simulink model "ASM_Traffic_V2X_Complete_Model_2"  (R2019a)
settings: Solver=ode1  StartTime=SIM.tstart.v  StopTime=Inf  FixedStep=SIM.StepSize.v  RelTol=1e-3
PostLoadFcn:
  | if any(exist('dsrtsu_mdlpostloadfcn', 'file') ~= 0), dsrtsu_mdlpostloadfcn('Execute', bdroot); end
  | try, asm_mdl_postloadfcn(bdroot, 'UpdateModel', 2200); catch, disp(lasterr); end,
undefined symbols (not defined in the file): _SensorPnts_1, _SensorPnts_13, _SensorPnts_17, _SensorPnts_21, _SensorPnts_25, _SensorPnts_29, _SensorPnts_33, _SensorPnts_37, _SensorPnts_41, _SensorPnts_45, _SensorPnts_49, _SensorPnts_5, _SensorPnts_53, _SensorPnts_57, _SensorPnts_9, _to_, CPT, G5A, ITS, MDL, rad, s_to_rpm, SIM
libraries: simulink x169, ASM_VehicleDynamics_lib x126, ASM_Traffic_lib x83, ASM_Utils_lib x49, mdbs x45, ASM_Environment_lib x17, dspindex x12, dsaV2xLibraryAux x10, dsmpblib x6, dsaV2xAsn1Library x4, dsaV2xLibrary x4, ASM_BrakeHydraulics_lib x4
(part 17 of 36)

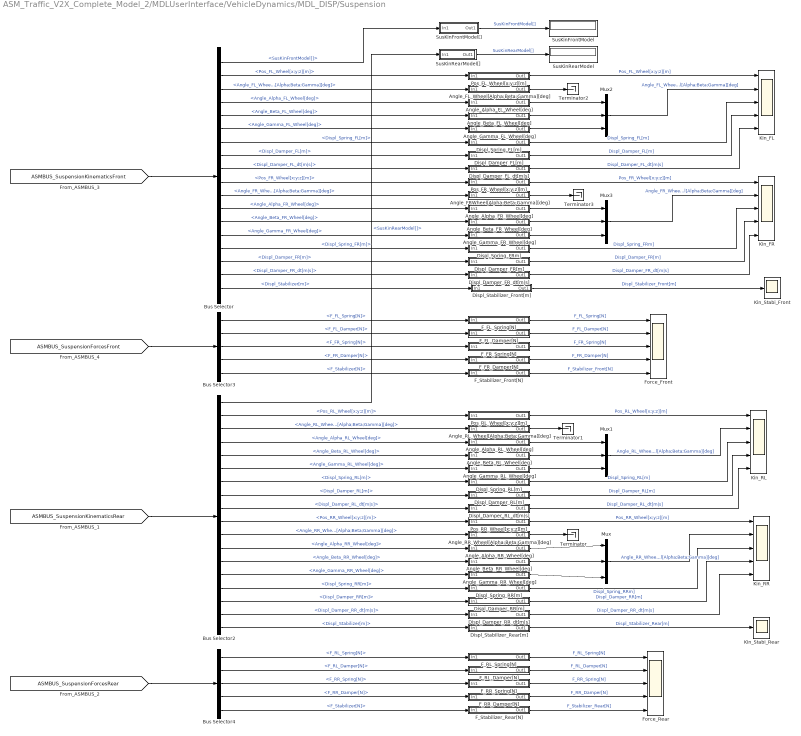
== system ASM_Traffic_V2X_Complete_Model_2/MDLUserInterface/VehicleDynamics/MDL_DISP/Suspension ==
  Angle_Alpha_FL_Wheel[deg] : Subsystem
      mask Display: disp('')
  Angle_Alpha_FR_Wheel[deg] : Subsystem
      mask Display: disp('')
  Angle_Alpha_RL_Wheel[deg] : Subsystem
      mask Display: disp('')
  Angle_Alpha_RR_Wheel[deg] : Subsystem
      mask Display: disp('')
  Angle_Beta_FL_Wheel[deg] : Subsystem
      mask Display: disp('')
  Angle_Beta_FR_Wheel[deg] : Subsystem
      mask Display: disp('')
  Angle_Beta_RL_Wheel[deg] : Subsystem
      mask Display: disp('')
  Angle_Beta_RR_Wheel[deg] : Subsystem
      mask Display: disp('')
  Angle_FL_Wheel[Alpha;Beta;Gamma][deg] : Subsystem
      mask Display: disp('')
  Angle_FRWheel[Alpha;Beta;Gamma][deg] : Subsystem
      mask Display: disp('')
  Angle_Gamma_FL_Wheel[deg] : Subsystem
      mask Display: disp('')
  Angle_Gamma_FR_Wheel[deg] : Subsystem
      mask Display: disp('')
  Angle_Gamma_RL_Wheel[deg] : Subsystem
      mask Display: disp('')
  Angle_Gamma_RR_Wheel[deg] : Subsystem
      mask Display: disp('')
  Angle_RL_Wheel[Alpha;Beta;Gamma][deg] : Subsystem
      mask Display: disp('')
  Angle_RR_Wheel[Alpha;Beta;Gamma][deg] : Subsystem
      mask Display: disp('')
  Bus Selector : BusSelector  OutputSignals=SusKinFrontModel[],Kinematics_Left.Position_Left.Pos_FL_Wheel[x;y;z][m],Kinematics_Left.Orientation_Left.Angle_FL_Wheel[Alpha;Beta;Gamma][deg],Kinematics_Left.Orientation_Left.Angle_FL_Wheel[Alpha;Beta;Gamma][deg].Angle_Alpha_FL_Wheel[deg],Kinematics_Left.Orientation_Left.Angle_FL_Wheel[Alpha;Beta;Gamma][deg].Angle_Beta_FL_Wheel[deg],Kinematics_Left.Orientation_Left.Angle_FL_Wheel[Alpha;Beta;Gamma][deg].Angle_Gamma_FL_Wheel[deg],Kinematics_Left.Spring_Left.Displ_Spring_FL[m],Kinematics_Left.Damper_Left.Displ_Damper_FL[m],Kinematics_Left.Damper_Left.Displ_Damper_FL_dt[m|s],Kinematics_Right.Position_Right.Pos_FR_Wheel[x;y;z][m],Kinematics_Right.Orientation_Right.Angle_FR_Wheel[Alpha;Beta;Gamma][deg],Kinematics_Right.Orientation_Right.Angle_FR_Wheel[Alpha;Beta;Gamma][deg].Angle_Alpha_FR_Wheel[deg],Kinematics_Right.Orientation_Right.Angle_FR_Wheel[Alpha;Beta;Gamma][deg].Angle_Beta_FR_Wheel[deg],Kinematics_Right.Orientation_Right.Angle_FR_Wheel[Alpha;Beta;Gamma][deg].Angle_Gamma_FR_Wheel[deg],Kinematics_Right.Spring_Right.Displ_Spring_FR[m],Kinematics_Right.Damper_Right.Displ_Damper_FR[m],Kinematics_Right.Damper_Right.Displ_Damper_FR_dt[m|s],Stabilizer.Displ_Stabilizer[m]
  Bus Selector2 : BusSelector  OutputSignals=SusKinRearModel[],Kinematics_Left.Position_Left.Pos_RL_Wheel[x;y;z][m],Kinematics_Left.Orientation_Left.Angle_RL_Wheel[Alpha;Beta;Gamma][deg],Kinematics_Left.Orientation_Left.Angle_RL_Wheel[Alpha;Beta;Gamma][deg].Angle_Alpha_RL_Wheel[deg],Kinematics_Left.Orientation_Left.Angle_RL_Wheel[Alpha;Beta;Gamma][deg].Angle_Beta_RL_Wheel[deg],Kinematics_Left.Orientation_Left.Angle_RL_Wheel[Alpha;Beta;Gamma][deg].Angle_Gamma_RL_Wheel[deg],Kinematics_Left.Spring_Left.Displ_Spring_RL[m],Kinematics_Left.Damper_Left.Displ_Damper_RL[m],Kinematics_Left.Damper_Left.Displ_Damper_RL_dt[m|s],Kinematics_Right.Position_Right.Pos_RR_Wheel[x;y;z][m],Kinematics_Right.Orientation_Right.Angle_RR_Wheel[Alpha;Beta;Gamma][deg],Kinematics_Right.Orientation_Right.Angle_RR_Wheel[Alpha;Beta;Gamma][deg].Angle_Alpha_RR_Wheel[deg],Kinematics_Right.Orientation_Right.Angle_RR_Wheel[Alpha;Beta;Gamma][deg].Angle_Beta_RR_Wheel[deg],Kinematics_Right.Orientation_Right.Angle_RR_Wheel[Alpha;Beta;Gamma][deg].Angle_Gamma_RR_Wheel[deg],Kinematics_Right.Spring_Right.Displ_Spring_RR[m],Kinematics_Right.Damper_Right.Displ_Damper_RR[m],Kinematics_Right.Damper_Right.Displ_Damper_RR_dt[m|s],Stabilizer.Displ_Stabilizer[m]
  Bus Selector3 : BusSelector  OutputSignals=F_FL_Spring[N],F_FL_Damper[N],F_FR_Spring[N],F_FR_Damper[N],F_Stabilizer[N]
  Bus Selector4 : BusSelector  OutputSignals=F_RL_Spring[N],F_RL_Damper[N],F_RR_Spring[N],F_RR_Damper[N],F_Stabilizer[N]
  Displ_Damper_FL[m] : Subsystem
      mask Display: disp('')
  Displ_Damper_FL_dt[m|s] : Subsystem
      mask Display: disp('')
  Displ_Damper_FR[m] : Subsystem
      mask Display: disp('')
  Displ_Damper_FR_dt[m|s] : Subsystem
      mask Display: disp('')
  Displ_Damper_RL[m] : Subsystem
      mask Display: disp('')
  Displ_Damper_RL_dt[m|s] : Subsystem
      mask Display: disp('')
  Displ_Damper_RR[m] : Subsystem
      mask Display: disp('')
  Displ_Damper_RR_dt[m|s] : Subsystem
      mask Display: disp('')
  Displ_Spring_FL[m] : Subsystem
      mask Display: disp('')
  Displ_Spring_FRm] : Subsystem
      mask Display: disp('')
  Displ_Spring_RL[m] : Subsystem
      mask Display: disp('')
  Displ_Spring_RR[m] : Subsystem
      mask Display: disp('')
  Displ_Stabilizer_Front[m] : Subsystem
      mask Display: disp('')
  Displ_Stabilizer_Rear[m] : Subsystem
      mask Display: disp('')
  F_FL_Damper[N] : Subsystem
      mask Display: disp('')
  F_FL_Spring[N] : Subsystem
      mask Display: disp('')
  F_FR_Damper[N] : Subsystem
      mask Display: disp('')
  F_FR_Spring[N] : Subsystem
      mask Display: disp('')
  F_RL_Damper[N] : Subsystem
      mask Display: disp('')
  F_RL_Spring[N] : Subsystem
      mask Display: disp('')
  F_RR_Damper[N] : Subsystem
      mask Display: disp('')
  F_RR_Spring[N] : Subsystem
      mask Display: disp('')
  F_Stabilizer_Front[N] : Subsystem
      mask Display: disp('')
  F_Stabilizer_Rear[N] : Subsystem
      mask Display: disp('')
  Force_Front : Scope  NumInputPorts=5
  Force_Rear : Scope  NumInputPorts=5
  Kin_FL : Scope  NumInputPorts=5
  Kin_FR : Scope  NumInputPorts=5
  Kin_RL : Scope  NumInputPorts=5
  Kin_RR : Scope  NumInputPorts=5
  Kin_Stabi_Front : Scope
  Kin_Stabi_Rear : Scope
  Mux{,1..3} (4 alike) : Mux  Inputs=3
  Pos_FL_Wheel[x;y;z][m] : Subsystem
      mask Display: disp('')
  Pos_FR_Wheel[x;y;z][m] : Subsystem
      mask Display: disp('')
  Pos_RL_Wheel[x;y;z][m] : Subsystem
      mask Display: disp('')
  Pos_RR_Wheel[x;y;z][m] : Subsystem
      mask Display: disp('')
  SusKinFrontModel : Display
  SusKinFrontModel[] : Subsystem
      mask Display: disp('')
  SusKinRearModel : Display
  SusKinRearModel[] : Subsystem
      mask Display: disp('')
  Terminator{,1..3} (4 alike) : Terminator
  wires:
  Bus Selector/14 -> Angle_Gamma_FR_Wheel[deg]/1(In1)  "<Angle_Gamma_FR_Wheel[deg]>"
  Bus Selector/13 -> Angle_Beta_FR_Wheel[deg]/1(In1)  "<Angle_Beta_FR_Wheel[deg]>"
  Bus Selector/12 -> Angle_Alpha_FR_Wheel[deg]/1(In1)  "<Angle_Alpha_FR_Wheel[deg]>"
  Angle_FRWheel[Alpha;Beta;Gamma][deg]/1(Out1) -> Terminator3/1
  Mux3/1 -> Kin_FR/2  "Angle_FR_Wheel[Alpha;Beta;Gamma][deg]"
  Angle_Gamma_FR_Wheel[deg]/1(Out1) -> Mux3/3
  Angle_Beta_FR_Wheel[deg]/1(Out1) -> Mux3/2
  Angle_Alpha_FR_Wheel[deg]/1(Out1) -> Mux3/1
  Bus Selector/15 -> Displ_Spring_FRm]/1(In1)  "<Displ_Spring_FR[m]>"
  Bus Selector/16 -> Displ_Damper_FR[m]/1(In1)  "<Displ_Damper_FR[m]>"
  Bus Selector/17 -> Displ_Damper_FR_dt[m|s]/1(In1)  "<Displ_Damper_FR_dt[m|s]>"
  Bus Selector/18 -> Displ_Stabilizer_Front[m]/1(In1)  "<Displ_Stabilizer[m]>"
  Bus Selector/11 -> Angle_FRWheel[Alpha;Beta;Gamma][deg]/1(In1)  "<Angle_FR_Wheel[Alpha;Beta;Gamma][deg]>"
  Bus Selector/10 -> Pos_FR_Wheel[x;y;z][m]/1(In1)  "<Pos_FR_Wheel[x;y;z][m]>"
  Bus Selector/9 -> Displ_Damper_FL_dt[m|s]/1(In1)  "<Displ_Damper_FL_dt[m|s]>"
  Bus Selector/8 -> Displ_Damper_FL[m]/1(In1)  "<Displ_Damper_FL[m]>"
  Bus Selector/7 -> Displ_Spring_FL[m]/1(In1)  "<Displ_Spring_FL[m]>"
  Bus Selector/6 -> Angle_Gamma_FL_Wheel[deg]/1(In1)  "<Angle_Gamma_FL_Wheel[deg]>"
  Bus Selector/5 -> Angle_Beta_FL_Wheel[deg]/1(In1)  "<Angle_Beta_FL_Wheel[deg]>"
  Bus Selector/4 -> Angle_Alpha_FL_Wheel[deg]/1(In1)  "<Angle_Alpha_FL_Wheel[deg]>"
  Mux2/1 -> Kin_FL/2  "Angle_FL_Wheel[Alpha;Beta;Gamma][deg]"
  Angle_FL_Wheel[Alpha;Beta;Gamma][deg]/1(Out1) -> Terminator2/1
  Angle_Gamma_FL_Wheel[deg]/1(Out1) -> Mux2/3
  Angle_Beta_FL_Wheel[deg]/1(Out1) -> Mux2/2
  Angle_Alpha_FL_Wheel[deg]/1(Out1) -> Mux2/1
  Bus Selector/3 -> Angle_FL_Wheel[Alpha;Beta;Gamma][deg]/1(In1)  "<Angle_FL_Wheel[Alpha;Beta;Gamma][deg]>"
  Angle_RL_Wheel[Alpha;Beta;Gamma][deg]/1(Out1) -> Terminator1/1
  Bus Selector2/6 -> Angle_Gamma_RL_Wheel[deg]/1(In1)  "<Angle_Gamma_RL_Wheel[deg]>"
  Bus Selector2/5 -> Angle_Beta_RL_Wheel[deg]/1(In1)  "<Angle_Beta_RL_Wheel[deg]>"
  Bus Selector2/4 -> Angle_Alpha_RL_Wheel[deg]/1(In1)  "<Angle_Alpha_RL_Wheel[deg]>"
  Mux1/1 -> Kin_RL/2  "Angle_RL_Wheel[Alpha;Beta;Gamma][deg]"
  Angle_Gamma_RL_Wheel[deg]/1(Out1) -> Mux1/3
  Angle_Beta_RL_Wheel[deg]/1(Out1) -> Mux1/2
  Angle_Alpha_RL_Wheel[deg]/1(Out1) -> Mux1/1
  Angle_RR_Wheel[Alpha;Beta;Gamma][deg]/1(Out1) -> Terminator/1
  Mux/1 -> Kin_RR/2  "Angle_RR_Wheel[Alpha;Beta;Gamma][deg]"
  Angle_Gamma_RR_Wheel[deg]/1(Out1) -> Mux/3
  Angle_Beta_RR_Wheel[deg]/1(Out1) -> Mux/2
  Angle_Alpha_RR_Wheel[deg]/1(Out1) -> Mux/1
  Bus Selector2/14 -> Angle_Gamma_RR_Wheel[deg]/1(In1)  "<Angle_Gamma_RR_Wheel[deg]>"
  Bus Selector2/13 -> Angle_Beta_RR_Wheel[deg]/1(In1)  "<Angle_Beta_RR_Wheel[deg]>"
  Bus Selector2/12 -> Angle_Alpha_RR_Wheel[deg]/1(In1)  "<Angle_Alpha_RR_Wheel[deg]>"
  Bus Selector2/1 -> SusKinRearModel[]/1(In1)  "<SusKinRearModel[]>"
  Bus Selector/1 -> SusKinFrontModel[]/1(In1)  "<SusKinFrontModel[]>"
  Bus Selector2/2 -> Pos_RL_Wheel[x;y;z][m]/1(In1)  "<Pos_RL_Wheel[x;y;z][m]>"
  Bus Selector/2 -> Pos_FL_Wheel[x;y;z][m]/1(In1)  "<Pos_FL_Wheel[x;y;z][m]>"
  [ASMBUS_SuspensionForcesRear] -> Bus Selector4/1
  [ASMBUS_SuspensionKinematicsRear] -> Bus Selector2/1
  [ASMBUS_SuspensionForcesFront] -> Bus Selector3/1
  [ASMBUS_SuspensionKinematicsFront] -> Bus Selector/1
  Bus Selector4/5 -> F_Stabilizer_Rear[N]/1(In1)  "<F_Stabilizer[N]>"
  Bus Selector4/4 -> F_RR_Damper[N]/1(In1)  "<F_RR_Damper[N]>"
  Bus Selector4/3 -> F_RR_Spring[N]/1(In1)  "<F_RR_Spring[N]>"
  Bus Selector4/2 -> F_RL_Damper[N]/1(In1)  "<F_RL_Damper[N]>"
  Bus Selector4/1 -> F_RL_Spring[N]/1(In1)  "<F_RL_Spring[N]>"
  Bus Selector2/18 -> Displ_Stabilizer_Rear[m]/1(In1)  "<Displ_Stabilizer[m]>"
  Bus Selector2/17 -> Displ_Damper_RR_dt[m|s]/1(In1)  "<Displ_Damper_RR_dt[m|s]>"
  Bus Selector2/16 -> Displ_Damper_RR[m]/1(In1)  "<Displ_Damper_RR[m]>"
  Bus Selector2/15 -> Displ_Spring_RR[m]/1(In1)  "<Displ_Spring_RR[m]>"
  Bus Selector2/11 -> Angle_RR_Wheel[Alpha;Beta;Gamma][deg]/1(In1)  "<Angle_RR_Wheel[Alpha;Beta;Gamma][deg]>"
  Bus Selector2/10 -> Pos_RR_Wheel[x;y;z][m]/1(In1)  "<Pos_RR_Wheel[x;y;z][m]>"
  Bus Selector2/9 -> Displ_Damper_RL_dt[m|s]/1(In1)  "<Displ_Damper_RL_dt[m|s]>"
  Bus Selector2/8 -> Displ_Damper_RL[m]/1(In1)  "<Displ_Damper_RL[m]>"
  Bus Selector2/7 -> Displ_Spring_RL[m]/1(In1)  "<Displ_Spring_RL[m]>"
  Bus Selector2/3 -> Angle_RL_Wheel[Alpha;Beta;Gamma][deg]/1(In1)  "<Angle_RL_Wheel[Alpha;Beta;Gamma][deg]>"
  Displ_Damper_RR_dt[m|s]/1(Out1) -> Kin_RR/5  "Displ_Damper_RR_dt[m|s]"
  Displ_Damper_RR[m]/1(Out1) -> Kin_RR/4  "Displ_Damper_RR[m]"
  Displ_Spring_RR[m]/1(Out1) -> Kin_RR/3  "Displ_Spring_RRm]"
  Pos_RR_Wheel[x;y;z][m]/1(Out1) -> Kin_RR/1  "Pos_RR_Wheel[x;y;z][m]"
  Displ_Stabilizer_Rear[m]/1(Out1) -> Kin_Stabi_Rear/1  "Displ_Stabilizer_Rear[m]"
  F_RL_Spring[N]/1(Out1) -> Force_Rear/1  "F_RL_Spring[N]"
  F_RL_Damper[N]/1(Out1) -> Force_Rear/2  "F_RL_Damper[N]"
  F_Stabilizer_Rear[N]/1(Out1) -> Force_Rear/5  "F_Stabilizer_Rear[N]"
  F_RR_Damper[N]/1(Out1) -> Force_Rear/4  "F_RR_Damper[N]"
  F_RR_Spring[N]/1(Out1) -> Force_Rear/3  "F_RR_Spring[N]"
  Displ_Damper_RL_dt[m|s]/1(Out1) -> Kin_RL/5  "Displ_Damper_RL_dt[m|s]"
  Displ_Damper_RL[m]/1(Out1) -> Kin_RL/4  "Displ_Damper_RL[m]"
  Displ_Spring_RL[m]/1(Out1) -> Kin_RL/3  "Displ_Spring_RL[m]"
  Pos_RL_Wheel[x;y;z][m]/1(Out1) -> Kin_RL/1  "Pos_RL_Wheel[x;y;z][m]"
  Displ_Damper_FR_dt[m|s]/1(Out1) -> Kin_FR/5  "Displ_Damper_FR_dt[m|s]"
  Displ_Damper_FR[m]/1(Out1) -> Kin_FR/4  "Displ_Damper_FR[m]"
  Displ_Spring_FRm]/1(Out1) -> Kin_FR/3  "Displ_Spring_FRm]"
  Pos_FR_Wheel[x;y;z][m]/1(Out1) -> Kin_FR/1  "Pos_FR_Wheel[x;y;z][m]"
  Displ_Stabilizer_Front[m]/1(Out1) -> Kin_Stabi_Front/1  "Displ_Stabilizer_Front[m]"
  F_FL_Spring[N]/1(Out1) -> Force_Front/1  "F_FL_Spring[N]"
  F_FL_Damper[N]/1(Out1) -> Force_Front/2  "F_FL_Damper[N]"
  F_Stabilizer_Front[N]/1(Out1) -> Force_Front/5  "F_Stabilizer_Front[N]"
  F_FR_Damper[N]/1(Out1) -> Force_Front/4  "F_FR_Damper[N]"
  F_FR_Spring[N]/1(Out1) -> Force_Front/3  "F_FR_Spring[N]"
  Bus Selector3/5 -> F_Stabilizer_Front[N]/1(In1)  "<F_Stabilizer[N]>"
  Bus Selector3/4 -> F_FR_Damper[N]/1(In1)  "<F_FR_Damper[N]>"
  Bus Selector3/3 -> F_FR_Spring[N]/1(In1)  "<F_FR_Spring[N]>"
  Bus Selector3/2 -> F_FL_Damper[N]/1(In1)  "<F_FL_Damper[N]>"
  Bus Selector3/1 -> F_FL_Spring[N]/1(In1)  "<F_FL_Spring[N]>"
  SusKinRearModel[]/1(Out1) -> SusKinRearModel/1  "SusKinRearModel[]"
  SusKinFrontModel[]/1(Out1) -> SusKinFrontModel/1  "SusKinFrontModel[]"
  Displ_Damper_FL_dt[m|s]/1(Out1) -> Kin_FL/5  "Displ_Damper_FL_dt[m|s]"
  Displ_Damper_FL[m]/1(Out1) -> Kin_FL/4  "Displ_Damper_FL[m]"
  Displ_Spring_FL[m]/1(Out1) -> Kin_FL/3  "Displ_Spring_FL[m]"
  Pos_FL_Wheel[x;y;z][m]/1(Out1) -> Kin_FL/1  "Pos_FL_Wheel[x;y;z][m]"

== system ASM_Traffic_V2X_Complete_Model_2/MDLUserInterface/VehicleDynamics/MDL_DISP/Tire ==
  Tire : Inport
  Bus Selector2 : BusSelector  OutputSignals=Tire_FL.ActiveTire.Slip_x_FL[],Tire_FR.ActiveTire.Slip_x_FR[],Tire_RL.ActiveTire.Slip_x_RL[],Tire_RR.ActiveTire.Slip_x_RR[],Tire_FL.ActiveTire.Slip_y_FL[],Tire_FR.ActiveTire.Slip_y_FR[],Tire_RL.ActiveTire.Slip_y_RL[],Tire_RR.ActiveTire.Slip_y_RR[],Tire_FL.ActiveTire.r_Dyn_FL_Tire[m],Tire_FR.ActiveTire.r_Dyn_FR_Tire[m],Tire_RL.ActiveTire.r_Dyn_RL_Tire[m],Tire_RR.ActiveTire.r_Dyn_RR_Tire[m],Tire_FL.ActiveTire.F_x_Dyn_FL_Tire_CoorSys_CP[N],Tire_FR.ActiveTire.F_x_Dyn_FR_Tire_CoorSys_CP[N],Tire_RL.ActiveTire.F_x_Dyn_RL_Tire_CoorSys_CP[N],Tire_RR.ActiveTire.F_x_Dyn_RR_Tire_CoorSys_CP[N],Tire_FL.ActiveTire.F_y_Dyn_FL_Tire_CoorSys_CP[N],Tire_FR.ActiveTire.F_y_Dyn_FR_Tire_CoorSys_CP[N],Tire_RL.ActiveTire.F_y_Dyn_RL_Tire_CoorSys_CP[N],Tire_RR.ActiveTire.F_y_Dyn_RR_Tire_CoorSys_CP[N],Tire_FL.ActiveTire.F_z_Dyn_FL_Tire_CoorSys_CP[N],Tire_FR.ActiveTire.F_z_Dyn_FR_Tire_CoorSys_CP[N],Tire_RL.ActiveTire.F_z_Dyn_RL_Tire_CoorSys_CP[N],Tire_RR.ActiveTire.F_z_Dyn_RR_Tire_CoorSys_CP[N],Tire_FL.ActiveTire.Trq_x_FL_CoorSys_CP[Nm],Tire_FR.ActiveTire.Trq_x_FR_CoorSys_CP[Nm],Tire_RL.ActiveTire.Trq_x_RL_CoorSys_CP[Nm],Tire_RR.ActiveTire.Trq_x_RR_CoorSys_CP[Nm],Tire_FL.ActiveTire.Trq_y_FL_CoorSys_W[Nm],Tire_FR.ActiveTire.Trq_y_FR_CoorSys_W[Nm],Tire_RL.ActiveTire.Trq_y_RL_CoorSys_W[Nm],Tire_RR.ActiveTire.Trq_y_RR_CoorSys_W[Nm],Tire_FL.ActiveTire.Trq_z_FL_CoorSys_CP[Nm],Tire_FR.ActiveTire.Trq_z_FR_CoorSys_CP[Nm],Tire_RL.ActiveTire.Trq_z_RL_CoorSys_CP[Nm],Tire_RR.ActiveTire.Trq_z_RR_CoorSys_CP[Nm],Tire_FL.ActiveTire.v_Circumf_Dyn_FL_Wheel[km|h],Tire_FR.ActiveTire.v_Circumf_Dyn_FR_Wheel[km|h],Tire_RL.ActiveTire.v_Circumf_Dyn_RL_Wheel[km|h],Tire_RR.ActiveTire.v_Circumf_Dyn_RR_Wheel[km|h]
  DynamicRadius : Scope  NumInputPorts=4
  F_x_Dyn_FL_Tire_CoorSys_CP[N] : Subsystem
      mask Display: disp('')
  F_x_Dyn_FR_Tire_CoorSys_CP[N] : Subsystem
      mask Display: disp('')
  F_x_Dyn_RL_Tire_CoorSys_CP[N] : Subsystem
      mask Display: disp('')
  F_x_Dyn_RR_Tire_CoorSys_CP[N] : Subsystem
      mask Display: disp('')
  F_y_Dyn_FL_Tire_CoorSys_CP[N] : Subsystem
      mask Display: disp('')
  F_y_Dyn_FR_Tire_CoorSys_CP[N] : Subsystem
      mask Display: disp('')
  F_y_Dyn_RL_Tire_CoorSys_CP[N] : Subsystem
      mask Display: disp('')
  F_y_Dyn_RR_Tire_CoorSys_CP[N] : Subsystem
      mask Display: disp('')
  F_z_Dyn_FL_Tire_CoorSys_CP[N] : Subsystem
      mask Display: disp('')
  F_z_Dyn_FR_Tire_CoorSys_CP[N] : Subsystem
      mask Display: disp('')
  F_z_Dyn_RL_Tire_CoorSys_CP[N] : Subsystem
      mask Display: disp('')
  F_z_Dyn_RR_Tire_CoorSys_CP[N] : Subsystem
      mask Display: disp('')
  Mux{,1..7} (8 alike) : Mux
  Slip : Scope  NumInputPorts=2
  Slip_x_FL[] : Subsystem
      mask Display: disp('')
  Slip_x_FR[] : Subsystem
      mask Display: disp('')
  Slip_x_RL[] : Subsystem
      mask Display: disp('')
  Slip_x_RR[] : Subsystem
      mask Display: disp('')
  Slip_y_FL[] : Subsystem
      mask Display: disp('')
  Slip_y_FR[] : Subsystem
      mask Display: disp('')
  Slip_y_RL[] : Subsystem
      mask Display: disp('')
  Slip_y_RR[] : Subsystem
      mask Display: disp('')
  TireCircumfSpeed : Scope  NumInputPorts=4
  TireForce : Scope  NumInputPorts=3
  TireTorque : Scope  NumInputPorts=3
  Trq_x_FL_CoorSys_CP[Nm] : Subsystem
      mask Display: disp('')
  Trq_x_FR_CoorSys_CP[Nm] : Subsystem
      mask Display: disp('')
  Trq_x_RL_CoorSys_CP[Nm] : Subsystem
      mask Display: disp('')
  Trq_x_RR_CoorSys_CP[Nm] : Subsystem
      mask Display: disp('')
  Trq_y_FL_CoorSys_W[Nm] : Subsystem
      mask Display: disp('')
  Trq_y_FR_CoorSys_W[Nm] : Subsystem
      mask Display: disp('')
  Trq_y_RL_CoorSys_W[Nm] : Subsystem
      mask Display: disp('')
  Trq_y_RR_CoorSys_W[Nm] : Subsystem
      mask Display: disp('')
  Trq_z_FL_CoorSys_CP[Nm] : Subsystem
      mask Display: disp('')
  Trq_z_FR_CoorSys_CP[Nm] : Subsystem
      mask Display: disp('')
  Trq_z_RL_CoorSys_CP[Nm] : Subsystem
      mask Display: disp('')
  Trq_z_RR_CoorSys_CP[Nm] : Subsystem
      mask Display: disp('')
  r_Dyn_FL_Tire[m] : Subsystem
      mask Display: disp('')
  r_Dyn_FR_Tire[m] : Subsystem
      mask Display: disp('')
  r_Dyn_RL_Tire[m] : Subsystem
      mask Display: disp('')
  r_Dyn_RR_Tire[m] : Subsystem
      mask Display: disp('')
  v_Circumf_Dyn_FL_Wheel[km|h] : Subsystem
      mask Display: disp('')
  v_Circumf_Dyn_FR_Wheel[km|h] : Subsystem
      mask Display: disp('')
  v_Circumf_Dyn_RL_Wheel[km|h] : Subsystem
      mask Display: disp('')
  v_Circumf_Dyn_RR_Wheel[km|h] : Subsystem
      mask Display: disp('')
  wires:
  Mux7/1 -> Slip/2  "Slip_y[]"
  Mux6/1 -> Slip/1  "Slip_x[]"
  Mux5/1 -> TireTorque/3  "Trq_z[Nm]"
  Mux3/1 -> TireTorque/2  "Trq_y[Nm]"
  Mux4/1 -> TireTorque/1  "Trq_x[Nm]"
  Mux2/1 -> TireForce/3  "F_z[N]"
  Mux/1 -> TireForce/2  "F_y[N]"
  Mux1/1 -> TireForce/1  "F_x[N]"
  Tire/1 -> Bus Selector2/1
  Slip_x_FL[]/1(Out1) -> Mux6/1  "Slip_x_FL[]"
  Slip_x_FR[]/1(Out1) -> Mux6/2  "Slip_x_FR[]"
  Slip_x_RL[]/1(Out1) -> Mux6/3  "Slip_x_RL[]"
  Slip_x_RR[]/1(Out1) -> Mux6/4  "Slip_x_RR[]"
  Slip_y_FL[]/1(Out1) -> Mux7/1  "Slip_y_FL[]"
  Slip_y_FR[]/1(Out1) -> Mux7/2  "Slip_y_FR[]"
  Slip_y_RL[]/1(Out1) -> Mux7/3  "Slip_y_RL[]"
  Slip_y_RR[]/1(Out1) -> Mux7/4  "Slip_y_RR[]"
  Bus Selector2/1 -> Slip_x_FL[]/1(In1)  "<Slip_x_FL[]>"
  Bus Selector2/2 -> Slip_x_FR[]/1(In1)  "<Slip_x_FR[]>"
  Bus Selector2/3 -> Slip_x_RL[]/1(In1)  "<Slip_x_RL[]>"
  Bus Selector2/4 -> Slip_x_RR[]/1(In1)  "<Slip_x_RR[]>"
  Bus Selector2/5 -> Slip_y_FL[]/1(In1)  "<Slip_y_FL[]>"
  Bus Selector2/6 -> Slip_y_FR[]/1(In1)  "<Slip_y_FR[]>"
  Bus Selector2/7 -> Slip_y_RL[]/1(In1)  "<Slip_y_RL[]>"
  Bus Selector2/8 -> Slip_y_RR[]/1(In1)  "<Slip_y_RR[]>"
  Trq_x_FL_CoorSys_CP[Nm]/1(Out1) -> Mux4/1  "Trq_x_FL_CoorSys_CP[Nm]"
  Trq_x_FR_CoorSys_CP[Nm]/1(Out1) -> Mux4/2  "Trq_x_FR_CoorSys_CP[Nm]"
  Trq_x_RL_CoorSys_CP[Nm]/1(Out1) -> Mux4/3  "Trq_x_RL_CoorSys_CP[Nm]"
  Trq_x_RR_CoorSys_CP[Nm]/1(Out1) -> Mux4/4  "Trq_x_RR_CoorSys_CP[Nm]"
  Trq_y_FL_CoorSys_W[Nm]/1(Out1) -> Mux3/1  "Trq_y_FL_CoorSys_W[Nm]"
  Trq_y_FR_CoorSys_W[Nm]/1(Out1) -> Mux3/2  "Trq_y_FR_CoorSys_W[Nm]"
  Trq_y_RL_CoorSys_W[Nm]/1(Out1) -> Mux3/3  "Trq_y_RL_CoorSys_W[Nm]"
  Trq_y_RR_CoorSys_W[Nm]/1(Out1) -> Mux3/4  "Trq_y_RR_CoorSys_W[Nm]"
  Trq_z_FL_CoorSys_CP[Nm]/1(Out1) -> Mux5/1  "Trq_z_FL_CoorSys_CP[Nm]"
  Trq_z_FR_CoorSys_CP[Nm]/1(Out1) -> Mux5/2  "Trq_z_FR_CoorSys_CP[Nm]"
  Trq_z_RL_CoorSys_CP[Nm]/1(Out1) -> Mux5/3  "Trq_z_RL_CoorSys_CP[Nm]"
  Trq_z_RR_CoorSys_CP[Nm]/1(Out1) -> Mux5/4  "Trq_z_RR_CoorSys_CP[Nm]"
  F_x_Dyn_FL_Tire_CoorSys_CP[N]/1(Out1) -> Mux1/1  "F_x_Dyn_FL_Tire_CoorSys_CP[N]"
  F_x_Dyn_FR_Tire_CoorSys_CP[N]/1(Out1) -> Mux1/2  "F_x_Dyn_FR_Tire_CoorSys_CP[N]"
  F_x_Dyn_RL_Tire_CoorSys_CP[N]/1(Out1) -> Mux1/3  "F_x_Dyn_RL_Tire_CoorSys_CP[N]"
  F_x_Dyn_RR_Tire_CoorSys_CP[N]/1(Out1) -> Mux1/4  "F_x_Dyn_RR_Tire_CoorSys_CP[N]"
  F_y_Dyn_FL_Tire_CoorSys_CP[N]/1(Out1) -> Mux/1  "F_y_Dyn_FL_Tire_CoorSys_CP[N]"
  F_y_Dyn_FR_Tire_CoorSys_CP[N]/1(Out1) -> Mux/2  "F_y_Dyn_FR_Tire_CoorSys_CP[N]"
  F_y_Dyn_RL_Tire_CoorSys_CP[N]/1(Out1) -> Mux/3  "F_y_Dyn_RL_Tire_CoorSys_CP[N]"
  F_y_Dyn_RR_Tire_CoorSys_CP[N]/1(Out1) -> Mux/4  "F_y_Dyn_RR_Tire_CoorSys_CP[N]"
  F_z_Dyn_FL_Tire_CoorSys_CP[N]/1(Out1) -> Mux2/1  "F_z_Dyn_FL_Tire_CoorSys_CP[N]"
  F_z_Dyn_FR_Tire_CoorSys_CP[N]/1(Out1) -> Mux2/2  "F_z_Dyn_FR_Tire_CoorSys_CP[N]"
  F_z_Dyn_RL_Tire_CoorSys_CP[N]/1(Out1) -> Mux2/3  "F_z_Dyn_RL_Tire_CoorSys_CP[N]"
  F_z_Dyn_RR_Tire_CoorSys_CP[N]/1(Out1) -> Mux2/4  "F_z_Dyn_RR_Tire_CoorSys_CP[N]"
  v_Circumf_Dyn_FL_Wheel[km|h]/1(Out1) -> TireCircumfSpeed/1  "v_Circumf_Dyn_FL_Wheel[km|h]"
  v_Circumf_Dyn_FR_Wheel[km|h]/1(Out1) -> TireCircumfSpeed/2  "v_Circumf_Dyn_FR_Wheel[km|h]"
  v_Circumf_Dyn_RL_Wheel[km|h]/1(Out1) -> TireCircumfSpeed/3  "v_Circumf_Dyn_RL_Wheel[km|h]"
  v_Circumf_Dyn_RR_Wheel[km|h]/1(Out1) -> TireCircumfSpeed/4  "v_Circumf_Dyn_RR_Wheel[km|h]"
  r_Dyn_FL_Tire[m]/1(Out1) -> DynamicRadius/1  "r_Dyn_FL_Tire[m]"
  r_Dyn_FR_Tire[m]/1(Out1) -> DynamicRadius/2  "r_Dyn_FR_Tire[m]"
  r_Dyn_RL_Tire[m]/1(Out1) -> DynamicRadius/3  "r_Dyn_RL_Tire[m]"
  r_Dyn_RR_Tire[m]/1(Out1) -> DynamicRadius/4  "r_Dyn_RR_Tire[m]"
  Bus Selector2/9 -> r_Dyn_FL_Tire[m]/1(In1)  "<r_Dyn_FL_Tire[m]>"
  Bus Selector2/10 -> r_Dyn_FR_Tire[m]/1(In1)  "<r_Dyn_FR_Tire[m]>"
  Bus Selector2/11 -> r_Dyn_RL_Tire[m]/1(In1)  "<r_Dyn_RL_Tire[m]>"
  Bus Selector2/12 -> r_Dyn_RR_Tire[m]/1(In1)  "<r_Dyn_RR_Tire[m]>"
  Bus Selector2/13 -> F_x_Dyn_FL_Tire_CoorSys_CP[N]/1(In1)  "<F_x_Dyn_FL_Tire_CoorSys_CP[N]>"
  Bus Selector2/14 -> F_x_Dyn_FR_Tire_CoorSys_CP[N]/1(In1)  "<F_x_Dyn_FR_Tire_CoorSys_CP[N]>"
  Bus Selector2/15 -> F_x_Dyn_RL_Tire_CoorSys_CP[N]/1(In1)  "<F_x_Dyn_RL_Tire_CoorSys_CP[N]>"
  Bus Selector2/16 -> F_x_Dyn_RR_Tire_CoorSys_CP[N]/1(In1)  "<F_x_Dyn_RR_Tire_CoorSys_CP[N]>"
  Bus Selector2/17 -> F_y_Dyn_FL_Tire_CoorSys_CP[N]/1(In1)  "<F_y_Dyn_FL_Tire_CoorSys_CP[N]>"
  Bus Selector2/18 -> F_y_Dyn_FR_Tire_CoorSys_CP[N]/1(In1)  "<F_y_Dyn_FR_Tire_CoorSys_CP[N]>"
  Bus Selector2/19 -> F_y_Dyn_RL_Tire_CoorSys_CP[N]/1(In1)  "<F_y_Dyn_RL_Tire_CoorSys_CP[N]>"
  Bus Selector2/20 -> F_y_Dyn_RR_Tire_CoorSys_CP[N]/1(In1)  "<F_y_Dyn_RR_Tire_CoorSys_CP[N]>"
  Bus Selector2/21 -> F_z_Dyn_FL_Tire_CoorSys_CP[N]/1(In1)  "<F_z_Dyn_FL_Tire_CoorSys_CP[N]>"
  Bus Selector2/22 -> F_z_Dyn_FR_Tire_CoorSys_CP[N]/1(In1)  "<F_z_Dyn_FR_Tire_CoorSys_CP[N]>"
  Bus Selector2/23 -> F_z_Dyn_RL_Tire_CoorSys_CP[N]/1(In1)  "<F_z_Dyn_RL_Tire_CoorSys_CP[N]>"
  Bus Selector2/24 -> F_z_Dyn_RR_Tire_CoorSys_CP[N]/1(In1)  "<F_z_Dyn_RR_Tire_CoorSys_CP[N]>"
  Bus Selector2/25 -> Trq_x_FL_CoorSys_CP[Nm]/1(In1)  "<Trq_x_FL_CoorSys_CP[Nm]>"
  Bus Selector2/26 -> Trq_x_FR_CoorSys_CP[Nm]/1(In1)  "<Trq_x_FR_CoorSys_CP[Nm]>"
  Bus Selector2/27 -> Trq_x_RL_CoorSys_CP[Nm]/1(In1)  "<Trq_x_RL_CoorSys_CP[Nm]>"
  Bus Selector2/28 -> Trq_x_RR_CoorSys_CP[Nm]/1(In1)  "<Trq_x_RR_CoorSys_CP[Nm]>"
  Bus Selector2/29 -> Trq_y_FL_CoorSys_W[Nm]/1(In1)  "<Trq_y_FL_CoorSys_W[Nm]>"
  Bus Selector2/30 -> Trq_y_FR_CoorSys_W[Nm]/1(In1)  "<Trq_y_FR_CoorSys_W[Nm]>"
  Bus Selector2/31 -> Trq_y_RL_CoorSys_W[Nm]/1(In1)  "<Trq_y_RL_CoorSys_W[Nm]>"
  Bus Selector2/32 -> Trq_y_RR_CoorSys_W[Nm]/1(In1)  "<Trq_y_RR_CoorSys_W[Nm]>"
  Bus Selector2/33 -> Trq_z_FL_CoorSys_CP[Nm]/1(In1)  "<Trq_z_FL_CoorSys_CP[Nm]>"
  Bus Selector2/34 -> Trq_z_FR_CoorSys_CP[Nm]/1(In1)  "<Trq_z_FR_CoorSys_CP[Nm]>"
  Bus Selector2/35 -> Trq_z_RL_CoorSys_CP[Nm]/1(In1)  "<Trq_z_RL_CoorSys_CP[Nm]>"
  Bus Selector2/36 -> Trq_z_RR_CoorSys_CP[Nm]/1(In1)  "<Trq_z_RR_CoorSys_CP[Nm]>"
  Bus Selector2/37 -> v_Circumf_Dyn_FL_Wheel[km|h]/1(In1)  "<v_Circumf_Dyn_FL_Wheel[km|h]>"
  Bus Selector2/38 -> v_Circumf_Dyn_FR_Wheel[km|h]/1(In1)  "<v_Circumf_Dyn_FR_Wheel[km|h]>"
  Bus Selector2/39 -> v_Circumf_Dyn_RL_Wheel[km|h]/1(In1)  "<v_Circumf_Dyn_RL_Wheel[km|h]>"
  Bus Selector2/40 -> v_Circumf_Dyn_RR_Wheel[km|h]/1(In1)  "<v_Circumf_Dyn_RR_Wheel[km|h]>"

== system ASM_Traffic_V2X_Complete_Model_2/MDLUserInterface/VehicleDynamics/MDL_DISP/Velocities ==
  Velocities : Inport
  Angle_SideSlip_Vehicle[deg] : Subsystem
      mask Display: disp('')
  AngularVelocities : Scope  NumInputPorts=3
  Bus Selector2 : BusSelector  OutputSignals=Vehicle.Linear.v_Vehicle_CoG[x;y;z][km|h].v_x_Vehicle_CoG[km|h],Vehicle.Linear.v_Vehicle_CoG[x;y;z][km|h].v_y_Vehicle_CoG[km|h],Vehicle.Linear.v_Vehicle_CoG[x;y;z][km|h].v_z_Vehicle_CoG[km|h],Vehicle.Linear.Angle_SideSlip_Vehicle[deg],Vehicle.Angular.w_Vehicle_CoG[x;y;z][deg|s].RollRate_Vehicle_CoG[deg|s],Vehicle.Angular.w_Vehicle_CoG[x;y;z][deg|s].PitchRate_Vehicle_CoG[deg|s],Vehicle.Angular.w_Vehicle_CoG[x;y;z][deg|s].YawRate_Vehicle_CoG[deg|s]
  PitchRate_Vehicle_CoG[deg|s] : Subsystem
      mask Display: disp('')
  RollRate_Vehicle_CoG[deg|s] : Subsystem
      mask Display: disp('')
  TransVelocities : Scope  NumInputPorts=4
  YawRate_Vehicle_CoG[deg|s] : Subsystem
      mask Display: disp('')
  v_x_Vehicle_CoG[km|h] : Subsystem
      mask Display: disp('')
  v_y_Vehicle_CoG[km|h] : Subsystem
      mask Display: disp('')
  v_z_Vehicle_CoG[km|h] : Subsystem
      mask Display: disp('')
  wires:
  Velocities/1 -> Bus Selector2/1
  RollRate_Vehicle_CoG[deg|s]/1(Out1) -> AngularVelocities/1  "RollRate_Vehicle_CoG[deg|s]"
  PitchRate_Vehicle_CoG[deg|s]/1(Out1) -> AngularVelocities/2  "PitchRate_Vehicle_CoG[deg|s]"
  YawRate_Vehicle_CoG[deg|s]/1(Out1) -> AngularVelocities/3  "YawRate_Vehicle_CoG[deg|s]"
  v_x_Vehicle_CoG[km|h]/1(Out1) -> TransVelocities/1  "v_x_Vehicle_CoG[km|h]"
  v_y_Vehicle_CoG[km|h]/1(Out1) -> TransVelocities/2  "v_y_Vehicle_CoG[km|h]"
  v_z_Vehicle_CoG[km|h]/1(Out1) -> TransVelocities/3  "v_z_Vehicle_CoG[km|h]"
  Angle_SideSlip_Vehicle[deg]/1(Out1) -> TransVelocities/4  "Angle_SideSlip_Vehicle[deg]"
  Bus Selector2/1 -> v_x_Vehicle_CoG[km|h]/1(In1)  "<v_x_Vehicle_CoG[km|h]>"
  Bus Selector2/2 -> v_y_Vehicle_CoG[km|h]/1(In1)  "<v_y_Vehicle_CoG[km|h]>"
  Bus Selector2/3 -> v_z_Vehicle_CoG[km|h]/1(In1)  "<v_z_Vehicle_CoG[km|h]>"
  Bus Selector2/4 -> Angle_SideSlip_Vehicle[deg]/1(In1)  "<Angle_SideSlip_Vehicle[deg]>"
  Bus Selector2/5 -> RollRate_Vehicle_CoG[deg|s]/1(In1)  "<RollRate_Vehicle_CoG[deg|s]>"
  Bus Selector2/6 -> PitchRate_Vehicle_CoG[deg|s]/1(In1)  "<PitchRate_Vehicle_CoG[deg|s]>"
  Bus Selector2/7 -> YawRate_Vehicle_CoG[deg|s]/1(In1)  "<YawRate_Vehicle_CoG[deg|s]>"

== system ASM_Traffic_V2X_Complete_Model_2/MDLUserInterface/VehicleDynamics/MDL_DISP/WheelSpeeds ==
  WheelSpeeds : Inport
  Bus Selector2 : BusSelector  OutputSignals=WheelSpeed.omega_FL_Wheel[rad|s],WheelSpeed.omega_FR_Wheel[rad|s],WheelSpeed.omega_RL_Wheel[rad|s],WheelSpeed.omega_RR_Wheel[rad|s]
  WheelSpeeds1 : Scope  NumInputPorts=4
  omega_FL_Wheel[rad|s] : Subsystem
      mask Display: disp('')
  omega_FR_Wheel[rad|s] : Subsystem
      mask Display: disp('')
  omega_RL_Wheel[rad|s] : Subsystem
      mask Display: disp('')
  omega_RR_Wheel[rad|s] : Subsystem
      mask Display: disp('')
  wires:
  omega_RR_Wheel[rad|s]/1(Out1) -> WheelSpeeds1/4  "omega_RR_Wheel[rad|s]"
  Bus Selector2/4 -> omega_RR_Wheel[rad|s]/1(In1)  "<omega_RR_Wheel[rad|s]>"
  omega_RL_Wheel[rad|s]/1(Out1) -> WheelSpeeds1/3  "omega_RL_Wheel[rad|s]"
  Bus Selector2/3 -> omega_RL_Wheel[rad|s]/1(In1)  "<omega_RL_Wheel[rad|s]>"
  omega_FR_Wheel[rad|s]/1(Out1) -> WheelSpeeds1/2  "omega_FR_Wheel[rad|s]"
  Bus Selector2/2 -> omega_FR_Wheel[rad|s]/1(In1)  "<omega_FR_Wheel[rad|s]>"
  omega_FL_Wheel[rad|s]/1(Out1) -> WheelSpeeds1/1  "omega_FL_Wheel[rad|s]"
  Bus Selector2/1 -> omega_FL_Wheel[rad|s]/1(In1)  "<omega_FL_Wheel[rad|s]>"
  WheelSpeeds/1 -> Bus Selector2/1

== system ASM_Traffic_V2X_Complete_Model_2/MDLUserInterface/VehicleDynamics/MDL_PAR/BrakeHydraulics_DistributionPattern_Switch ==
  Sw_DistributionPattern[1X|2II] : Constant
  tag scope: TAG_Sw_DistributionPattern=global
  wires:
  Sw_DistributionPattern[1X|2II]/1 -> [TAG_Sw_DistributionPattern]

== system ASM_Traffic_V2X_Complete_Model_2/MDLUserInterface/VehicleDynamics/MDL_PAR/Suspension_Inits ==
  Bus Creator1 : BusCreator  Inputs=2
  Mux : Mux
  Mux2 : Mux
  z_FL_Init[m] : Constant  Value=0  VectorParams1D=off
  z_FL_Init_dt[m|s] : Constant  Value=0  VectorParams1D=off
  z_FR_Init[m] : Constant  Value=0  VectorParams1D=off
  z_FR_Init_dt[m|s] : Constant  Value=0  VectorParams1D=off
  z_RL_Init[m] : Constant  Value=0  VectorParams1D=off
  z_RL_Init_dt[m|s] : Constant  Value=0  VectorParams1D=off
  z_RR_Init[m] : Constant  Value=0  VectorParams1D=off
  z_RR_Init_dt[m|s] : Constant  Value=0  VectorParams1D=off
  tag scope: TAG_Suspension_Init=global
  wires:
  Mux2/1 -> Bus Creator1/1  "q_dt_Wheel_Init[:]"
  Mux/1 -> Bus Creator1/2  "q_Wheel_Init[:]"
  Bus Creator1/1 -> [TAG_Suspension_Init]
  z_FL_Init_dt[m|s]/1 -> Mux2/1
  z_FR_Init_dt[m|s]/1 -> Mux2/2
  z_RL_Init_dt[m|s]/1 -> Mux2/3
  z_RR_Init_dt[m|s]/1 -> Mux2/4
  z_FL_Init[m]/1 -> Mux/1
  z_FR_Init[m]/1 -> Mux/2
  z_RL_Init[m]/1 -> Mux/3
  z_RR_Init[m]/1 -> Mux/4

== system ASM_Traffic_V2X_Complete_Model_2/MDLUserInterface/VehicleDynamics/MDL_PAR/Tire_Switches ==
  Bus Creator1 : BusCreator  Inputs=2
  Sw_r_Tire[1:intern;2:extern] : Constant  VectorParams1D=off
  r_Tire_extern[m] : Constant  Value=0.31  VectorParams1D=off
  tag scope: TAG_Tire_Switches=global
  wires:
  Bus Creator1/1 -> [TAG_Tire_Switches]
  Sw_r_Tire[1:intern;2:extern]/1 -> Bus Creator1/1  "Sw_r_Tire[1:intern;2:extern]"
  r_Tire_extern[m]/1 -> Bus Creator1/2  "r_Tire_extern[m]"

== system ASM_Traffic_V2X_Complete_Model_2/IO/I//O_Subsystem/Bus Configuration (1) - In/Simulated ECUs/DrivekitCAN ==
  Input : Inport
  Drivekit : Subsystem
  _DrivekitCAN_ : BusCreator  Inputs=1
  DrivekitCAN : Outport
  wires:
  _DrivekitCAN_/1 -> DrivekitCAN/1  "DrivekitCAN"
  Drivekit/1(Drivekit) -> _DrivekitCAN_/1  "Drivekit"
  Input/1 -> Drivekit/1(Input)

== system ASM_Traffic_V2X_Complete_Model_2/IO/I//O_Subsystem/Bus Configuration (1) - Out/Simulated ECUs/DrivekitCAN ==
  DrivekitCAN : Inport
  Drivekit : Subsystem
  _DrivekitCAN_ : BusSelector  OutputSignals=Drivekit
  wires:
  DrivekitCAN/1 -> _DrivekitCAN_/1  "DrivekitCAN"
  _DrivekitCAN_/1 -> Drivekit/1(Drivekit)  "<Drivekit>"

== system ASM_Traffic_V2X_Complete_Model_2/IO/V2X_Subsystem/CAM-DENM_Message_Generation/DENM/Alternative_UDP2ControlPC_Directly ==
  Trigger : TriggerPort  VariantControl=Variant  PortDimensions=1
  Byte Pack : etargetslib/Byte Pack  datatypes={'uint32','uint32'}  byteAlign=1
      settings: SourceProductName=MATLAB Coder
  Byte Pack1 : etargetslib/Byte Pack  datatypes={['uint8'],'uint32','uint32','int32','int32'}  byteAlign=1
      settings: SourceProductName=MATLAB Coder
  Byte Pack2 : etargetslib/Byte Pack  datatypes={'uint16','uint8','uint8',['uint8']}  byteAlign=1
      settings: SourceProductName=MATLAB Coder
  Interface : Constant  Value=144  OutDataTypeStr=uint8
  Length : Constant  Value=130  OutDataTypeStr=uint16  LockScale=on
  Seconds1 : Constant  Value=0  OutDataTypeStr=uint32
  SentBytes : Display
  Status : Display
  UDP Transmit (2)_In1 : dsmpblib/Data Inport  Priority=10000
      settings: SourceProductName=dSPACE Model Interface Blockset
  UDP Transmit (2)_Out1 : dsmpblib/Data Outport  Priority=-10000
      settings: SourceProductName=dSPACE Model Interface Blockset
  Version : Constant  Value=4  OutDataTypeStr=uint8
  Width1 : Width
  distance2event1 : Constant  Value=500  OutDataTypeStr=uint32
  lat_event1 : Constant  Value=51074999  OutDataTypeStr=int32
  lon_event1 : Constant  Value=6148851  OutDataTypeStr=int32
  nanoseconds1 : Constant  Value=0  OutDataTypeStr=uint32
  triggerTimeOfMRM1 : Constant  Value=0  OutDataTypeStr=uint32
  wires:
  nanoseconds1/1 -> Byte Pack/2
  Width1/1 -> UDP Transmit (2)_Out1/2
  Seconds1/1 -> Byte Pack/1
  Interface/1 -> Byte Pack2/2
  Byte Pack2/1 -> UDP Transmit (2)_Out1/1, Width1/1
  triggerTimeOfMRM1/1 -> Byte Pack1/2
  Length/1 -> Byte Pack2/1
  UDP Transmit (2)_In1/1 -> Status/1
  distance2event1/1 -> Byte Pack1/3
  Version/1 -> Byte Pack2/3
  UDP Transmit (2)_In1/2 -> SentBytes/1
  Byte Pack/1 -> Byte Pack1/1
  Byte Pack1/1 -> Byte Pack2/4
  lon_event1/1 -> Byte Pack1/5
  lat_event1/1 -> Byte Pack1/4

== system ASM_Traffic_V2X_Complete_Model_2/IO/V2X_Subsystem/CAM-DENM_Message_Generation/DENM/Create_DENM ==
  dsaAsn1EncoderSfcn_BL1 : dsaV2xAsn1Library/dsaAsn1EncoderSfcn_BL1  xml=|  typeStr=DENM (ETSI EN 302 637-3 v1.2.1)  encDecType=2  sampleTime=-1  outBufferMaxLen=1800  maxSpacePerNumber=100
      | <DENM>
      |     <header>
      |         <protocolVersion>1</protocolVersion>
      |         <messageID>1</messageID>
      |         <stationID>5</stationID>
      |     </header>
      |     <denm>
      |         <management>
      |             <actionID>
      |                 <originatingStationID>61</originatingStationID>
      |                 <sequenceNumber>16504</sequenceNumber>
      |             </actionID>
      |             <detectionTime>517786000000</detectionTime>
      |             <referenceTime>517711000000</referenceTime>
      |             <eventPosition>
      |                 <latitude>510750187</latitude>
      |                 <longitude>61387357</longitude>
      |                 <positionConfidenceEllipse>
      |                     <semiMajorConfidence>500</semiMajorConfidence>
      |                     <semiMinorConfidence>400</semiMinorConfidence>
      |                     <semiMajorOrientation>10</semiMajorOrientation>
      |                 </positionConfidenceEllipse>
      |                 <altitude>
      |                     <altitudeValue>8000</altitudeValue>
      |                     <altitudeConfidence>
      |                         <alt-005-00/>
      |                     </altitudeConfidence>
      |                 </altitude>
      |             </eventPosition>
      |             <relevanceDistance>
      |                 <lessThan5km/>
      |             </relevanceDistance>
      |             <validityDuration>600</validityDuration>
      |             <stationType>78</stationType>
      |         </management>
      |         <situation>
      |             <informationQuality>1</informationQuality>
      |             <eventType>
      |                 <causeCode>3</causeCode>
      |                 <subCauseCode>0</subCauseCode>
      |             </eventType>
      |         </situation>
      |         <location>
      |             <eventSpeed>
      |                 <speedValue>0</speedValue>
      |                 <speedConfidence>1</speedConfidence>
      |             </eventSpeed>
      |             <eventPositionHeading>
      |                 <headingValue>2232</headingValue>
      |                 <headingConfidence>85</headingConfidence>
      |             </eventPositionHeading>
      |             <traces>
      |                 <PathHistory>
      |                     <PathPoint>
      |                         <pathPosition>
      |                             <deltaLatitude>-14842</deltaLatitude>
      |                             <deltaLongitude>-60138</deltaLongitude>
      |                             <deltaAltitude>-10002</deltaAltitude>
      |                         </pathPosition>
      |                         <pathDeltaTime>0</pathDeltaTime>
      |                     </PathPoint>
      |                 </PathHistory>
      |             </traces>
      |         </location>
      |     </denm>
      | </DENM>
      settings: AttributesFormatString=%<typeStr>  SourceProductName=dSPACE [SOL] V2X ASN.1 Blockset
  dsaV2xBusAdapter_a_BL2 : Subsystem  AncestorBlock=dsaV2xLibraryAux/dsaV2xBusAdapter_a_BL1
      mask Display: disp('V2X-Bus\nCreator');
  DENM1 : Outport
  wires:
  dsaAsn1EncoderSfcn_BL1/3 -> dsaV2xBusAdapter_a_BL2/3(Data)
  dsaAsn1EncoderSfcn_BL1/1 -> dsaV2xBusAdapter_a_BL2/1(Status)
  dsaAsn1EncoderSfcn_BL1/2 -> dsaV2xBusAdapter_a_BL2/2(Length)
  dsaV2xBusAdapter_a_BL2/1(V2X-Bus) -> DENM1/1

== system ASM_Traffic_V2X_Complete_Model_2/IO/V2X_Subsystem/CAM-DENM_Message_Generation/DENM/DENM_Encode ==
  DENM : Inport
  Trigger : TriggerPort  VariantControl=Variant  PortDimensions=1
  Compare To Zero : simulink/Logic and Bit Operations/Compare To Zero  relop===  OutDataTypeStr=boolean
  Data Type Conversion{1..4} (4 alike) : DataTypeConversion
  Enabled : Constant  OutDataTypeStr=Inherit: Inherit via back propagation
  Mux1 : Mux  Inputs=2
  Terminator1 : Terminator
  Terminator3 : Terminator
  dsa_BTP_and_GeoNetworking_Request_BL1 : dsaV2xLibrary/dsa_BTP_and_GeoNetworking_Request_BL1  btpType=BTP-B (non-interactive)  destinationPort=DENM  sourcePort=CAM  destinationPortInfo=0 (default)  packetTransportType=Topologically Scoped Brodcast (Single hop)  communicationProfile=ITS-G5A  securityProfile=C2XSEC_NONE  maximumPacketLifetime=5  maximumPacketLifetimeMode=disabled  repetitionInterval=250  repetitionIntervalMode=disabled  maximumRepetitionTime=5  maximumRepetitionTimeMode=disabled  maximumHopLimit=4  maximumHopLimitMode=disabled  scf=off  channelOffload=off  tcId=DENM  style=CohdaWireless MK5
      settings: SourceProductName=dSPACE [SOL] V2X Blockset
  dsa_generic_eth_udp_adapter_BL1 : dsaV2xLibraryAux/dsa_generic_eth_udp_adapter_BL1  style=SCALEXIO Ethernet Solution  direction=Tx  maxSize=1472
  OutputDENM : Outport
  wires:
  Enabled/1 -> dsa_generic_eth_udp_adapter_BL1/1
  dsa_BTP_and_GeoNetworking_Request_BL1/3 -> Data Type Conversion1/1
  dsa_BTP_and_GeoNetworking_Request_BL1/1 -> Compare To Zero/1
  Data Type Conversion4/1 -> dsa_generic_eth_udp_adapter_BL1/2
  dsa_BTP_and_GeoNetworking_Request_BL1/2 -> Data Type Conversion4/1
  Data Type Conversion3/1 -> Mux1/2
  Mux1/1 -> OutputDENM/1
  Compare To Zero/1 -> Terminator1/1
  Data Type Conversion2/1 -> Mux1/1
  dsa_generic_eth_udp_adapter_BL1/1 -> Terminator3/1
  dsa_generic_eth_udp_adapter_BL1/3 -> Data Type Conversion3/1
  dsa_generic_eth_udp_adapter_BL1/2 -> Data Type Conversion2/1
  Data Type Conversion1/1 -> dsa_generic_eth_udp_adapter_BL1/3
  DENM/1 -> dsa_BTP_and_GeoNetworking_Request_BL1/1

== system ASM_Traffic_V2X_Complete_Model_2/IO/V2X_Subsystem/CAM-DENM_Message_Generation/DENM/DENM_trigger_Conditions ==
  In1 : Inport
  AND : Logic  Inputs=3  IconShape=distinctive  AllPortsSameDT=off  OutDataTypeStr=boolean
  AND1 : Logic  IconShape=distinctive  AllPortsSameDT=off  OutDataTypeStr=boolean
  Bus Selector : BusSelector  OutputSignals=signal4.s_Veh_Road[m]
  Bus Selector1 : BusSelector  OutputSignals=signal4.s_Veh_Road[m]
  DENM_Switch : Constant
  Data Type Conversion : DataTypeConversion
  Data Type Conversion1 : DataTypeConversion
  Data Type Conversion2 : DataTypeConversion
  "Distance_to_NoADZone " : Display
  NoADZone_Start : Constant  Value=1000
  Pulse Generator : DiscretePulseGenerator  PulseType=Time based  Period=1  PulseWidth=90
  Relational Operator : RelationalOperator  OutDataTypeStr=boolean  RndMeth=Simplest
  Relational Operator1 : RelationalOperator  Operator=<=  OutDataTypeStr=boolean  RndMeth=Simplest
  Subtract : Sum  Inputs=+-
  TOR_Dist_1 : Constant  Value=500
  TOR_Dist_2 : Constant  Value=505
  s_Veh_Road[m] : Display
  Out1 : Outport
  wires:
  DENM_Switch/1 -> AND/1
  Pulse Generator/1 -> AND/2
  TOR_Dist_1/1 -> Relational Operator/2
  In1/1 -> Bus Selector1/1, Bus Selector/1
  Bus Selector/1 -> Relational Operator1/1, Relational Operator/1  "<s_Veh_Road[m]>"
  Data Type Conversion/1 -> AND/3
  AND/1 -> Out1/1
  Relational Operator/1 -> Data Type Conversion1/1
  TOR_Dist_2/1 -> Relational Operator1/2
  Relational Operator1/1 -> Data Type Conversion2/1
  Data Type Conversion1/1 -> AND1/1
  Data Type Conversion2/1 -> AND1/2
  AND1/1 -> Data Type Conversion/1
  Bus Selector1/1 -> s_Veh_Road[m]/1, Subtract/2  "<s_Veh_Road[m]>"
  NoADZone_Start/1 -> Subtract/1
  Subtract/1 -> "Distance_to_NoADZone "/1

== system ASM_Traffic_V2X_Complete_Model_2/IO/V2X_Subsystem/CAM-DENM_Message_Generation/DENM/UDP_Trigger ==
  In1 : Inport
  AND : Logic  IconShape=distinctive  AllPortsSameDT=off  OutDataTypeStr=boolean
  Bus Selector : BusSelector  OutputSignals=v_Total_Vehicle[km|h]
  Clock : Clock
  Relational Operator : RelationalOperator  Operator=<=  OutDataTypeStr=boolean  RndMeth=Simplest
  Relational Operator1 : RelationalOperator  OutDataTypeStr=boolean  RndMeth=Simplest
  SpeedCondition : Constant  Value=20
  TimeCondition : Constant  Value=5
  Out1 : Outport
  wires:
  SpeedCondition/1 -> Relational Operator/1
  In1/1 -> Bus Selector/1
  Bus Selector/1 -> Relational Operator/2  "<v_Total_Vehicle[km|h]>"
  Clock/1 -> Relational Operator1/1
  TimeCondition/1 -> Relational Operator1/2
  Relational Operator/1 -> AND/1
  Relational Operator1/1 -> AND/2
  AND/1 -> Out1/1

== system ASM_Traffic_V2X_Complete_Model_2/IO/V2X_Subsystem/CAM-DENM_Message_Generation/Fellow_CAM_1/CAM_Encode ==
  " CAM" : Inport
  Trigger : TriggerPort  VariantControl=Variant  PortDimensions=1
  Compare To Zero : simulink/Logic and Bit Operations/Compare To Zero  relop===  OutDataTypeStr=boolean
  Data Type Conversion{1..4} (4 alike) : DataTypeConversion
  Enabled : Constant  OutDataTypeStr=Inherit: Inherit via back propagation
  Terminator1 : Terminator
  Terminator3 : Terminator
  dsa_BTP_and_GeoNetworking_Request_BL3 : dsaV2xLibrary/dsa_BTP_and_GeoNetworking_Request_BL1  btpType=BTP-B (non-interactive)  destinationPort=CAM  sourcePort=CAM  destinationPortInfo=0 (default)  packetTransportType=Topologically Scoped Brodcast (Single hop)  communicationProfile=ITS-G5A  securityProfile=C2XSEC_NONE  maximumPacketLifetime=5  maximumPacketLifetimeMode=disabled  repetitionInterval=250  repetitionIntervalMode=disabled  maximumRepetitionTime=5  maximumRepetitionTimeMode=disabled  maximumHopLimit=1  maximumHopLimitMode=disabled  scf=off  channelOffload=off  tcId=CAM  style=CohdaWireless MK5
      settings: SourceProductName=dSPACE [SOL] V2X Blockset
  dsa_generic_eth_udp_adapter_BL1 : dsaV2xLibraryAux/dsa_generic_eth_udp_adapter_BL1  style=SCALEXIO Ethernet Solution  direction=Tx  maxSize=1472
  Data : Outport
  Bytes : Outport  Port=2
  wires:
  Compare To Zero/1 -> Terminator1/1
  dsa_BTP_and_GeoNetworking_Request_BL3/1 -> Compare To Zero/1
  Data Type Conversion3/1 -> Bytes/1
  " CAM"/1 -> dsa_BTP_and_GeoNetworking_Request_BL3/1
  Data Type Conversion2/1 -> Data/1
  Data Type Conversion1/1 -> dsa_generic_eth_udp_adapter_BL1/3
  dsa_BTP_and_GeoNetworking_Request_BL3/2 -> Data Type Conversion4/1
  Data Type Conversion4/1 -> dsa_generic_eth_udp_adapter_BL1/2
  dsa_BTP_and_GeoNetworking_Request_BL3/3 -> Data Type Conversion1/1
  dsa_generic_eth_udp_adapter_BL1/1 -> Terminator3/1
  dsa_generic_eth_udp_adapter_BL1/2 -> Data Type Conversion2/1
  dsa_generic_eth_udp_adapter_BL1/3 -> Data Type Conversion3/1
  Enabled/1 -> dsa_generic_eth_udp_adapter_BL1/1
